simulink library "groundStation000_cl"  (R2018b)
settings: Solver=VariableStepAuto  StartTime=0.0  StopTime=10.0  RelTol=1e-3
undefined symbols (not defined in the file): gndStnMmtArms, ini_platform_ang, ini_platform_vel, sim_param
libraries: eulAng2RotMat_ul x1, massSpringDamper_ul x1, tethersMoment_cl x1, thrAttachPtKinematics_ul x1
settings Model: Creator=M.Cobb  LastModifiedBy=mcobb

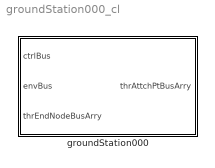
== system groundStation000_cl ==
  groundStation000 : Subsystem  mask{fixed=1, J=sim_param.platform_param.platform_Izz, b=sim_param.platform_param.platform_damping, posVec=[0 0 0], thrAttachPt=sim_param.tether_imp_nodes.R11_g, initAngPos=ini_platform_ang, initAngVel=ini_platform_vel}
      mask prompts: fixed "Free Spin Enable (==0 -> No Rotation, ~=0 -> Free Spinning)"; J "Rotational Inertia"; b "Damping coefficient"; posVec "Position Vector"; thrAttachPt "Tether attachment points"; initAngPos "Initial angle"; initAngVel "Inital angular velocity"
      mask DialogControl Container5 Prompt: Physical Parameters
      mask DialogControl Container3 Prompt: Tether attachment position vectors: platform frame
      mask DialogControl Container4 Prompt: Initial conditions

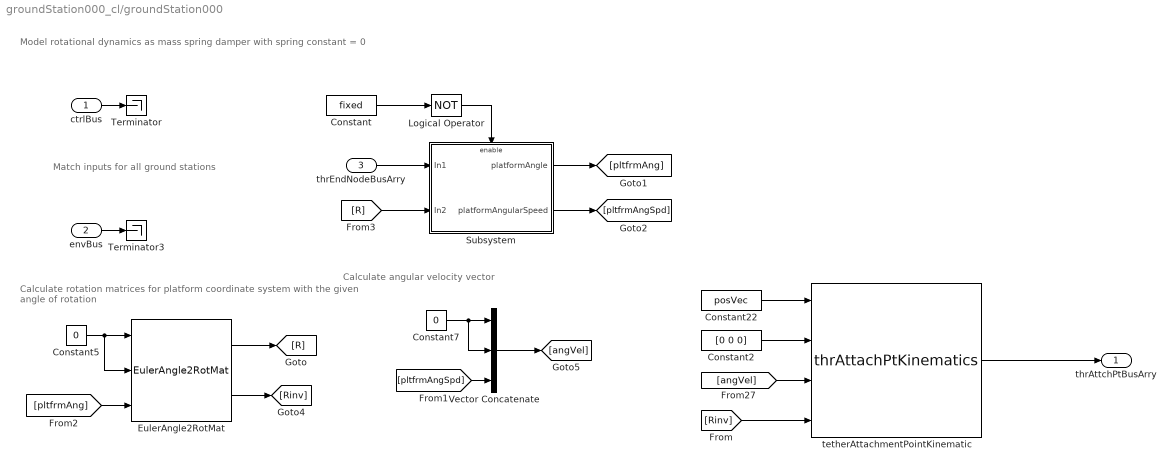
== system groundStation000_cl/groundStation000 ==
  note: Match inputs for all ground stations
  note: Calculate rotation matrices for platform coordinate
      | system with the given angle of rotation
  note: Calculate angular velocity vector
  note: Model rotational dynamics as mass spring damper with
      | spring constant = 0
  ctrlBus : Inport  OutDataTypeStr=Bus: ctrlBus
  envBus : Inport  Port=2  OutDataTypeStr=Bus: envBus
  thrEndNodeBusArry : Inport  Port=3
  Constant : Constant  Value=fixed
  Constant2 : Constant  Value=[0 0 0]
  Constant22 : Constant  Value=posVec
  Constant5 : Constant  Value=0
  Constant7 : Constant  Value=0
  EulerAngle2RotMat : eulAng2RotMat_ul/EulerAngle2RotMat  SystemSampleTime=-1
  Logical Operator : Logic  Operator=NOT  AllPortsSameDT=off  OutDataTypeStr=boolean
  Subsystem : Subsystem
  Terminator : Terminator
  Terminator3 : Terminator
  Vector Concatenate : Concatenate  NumInputs=3
  tetherAttachmentPointKinematic : thrAttachPtKinematics_ul/thrAttachPtKinematics  atchPts=thrAttachPt
  thrAttchPtBusArry : Outport
  wires:
  Constant5/1 -> EulerAngle2RotMat/2, EulerAngle2RotMat/1
  EulerAngle2RotMat/1 -> [R]
  EulerAngle2RotMat/2 -> [Rinv]
  Constant7/1 -> Vector Concatenate/1, Vector Concatenate/2
  Vector Concatenate/1 -> [angVel]
  tetherAttachmentPointKinematic/1 -> thrAttchPtBusArry/1
  Constant22/1 -> tetherAttachmentPointKinematic/1
  Constant2/1 -> tetherAttachmentPointKinematic/2
  [Rinv] -> tetherAttachmentPointKinematic/4
  [angVel] -> tetherAttachmentPointKinematic/3
  [pltfrmAngSpd] -> Vector Concatenate/3
  [pltfrmAng] -> EulerAngle2RotMat/3
  ctrlBus/1 -> Terminator/1
  envBus/1 -> Terminator3/1
  Constant/1 -> Logical Operator/1
  Logical Operator/1 -> Subsystem/Enable
  thrEndNodeBusArry/1 -> Subsystem/1(In1)
  [R] -> Subsystem/2(In2)
  Subsystem/1(platformAngle) -> [pltfrmAng]
  Subsystem/2(platformAngularSpeed) -> [pltfrmAngSpd]

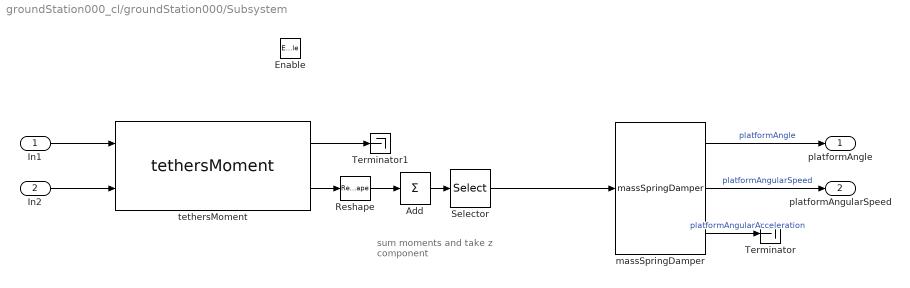
== system groundStation000_cl/groundStation000/Subsystem ==
  note: sum moments and
      | take z component
  In1 : Inport
  In2 : Inport  Port=2
  Enable : EnablePort
  Add : Sum  Inputs=+  CollapseMode=Specified dimension  CollapseDim=2
  Reshape : Reshape  OutputDimensionality=Customize  OutputDimensions=[3 numel(gndStnMmtArms)]
  Selector : Selector  InputPortWidth=3  IndexOptions=Index vector (dialog)  Indices=3  OutputSizes=1
  Terminator : Terminator
  Terminator1 : Terminator
  massSpringDamper : massSpringDamper_ul/massSpringDamper  m=J  b=b  k=0  x0=initAngPos  xDot0=initAngVel
  tethersMoment : tethersMoment_cl/tethersMoment  arms=thrAttachPt
  platformAngle : Outport  InitialOutput=initAngPos
  platformAngularSpeed : Outport  Port=2  InitialOutput=initAngVel
  wires:
  massSpringDamper/2 -> platformAngularSpeed/1  "platformAngularSpeed"
  Add/1 -> Selector/1
  Selector/1 -> massSpringDamper/1
  Reshape/1 -> Add/1
  tethersMoment/1 -> Terminator1/1
  tethersMoment/2 -> Reshape/1
  In1/1 -> tethersMoment/1
  In2/1 -> tethersMoment/2
  massSpringDamper/1 -> platformAngle/1  "platformAngle"
  massSpringDamper/3 -> Terminator/1  "platformAngularAcceleration"
